simulink model "AutoParkFollowingBehaviour"  (R2023b)
settings: Solver=VariableStepAuto  StartTime=0  StopTime=2000  RelTol=1e-3
values from neighbouring files (symbols this model uses):
  simStepSize = 0.1    [AutoParkScenarioScript.m]
undefined symbols (not defined in the file or in its folder): Defined, Ego, Lane, User
libraries: roadrunnerscenario x3
settings Model: Creator=darkh  LastModifiedBy=varun

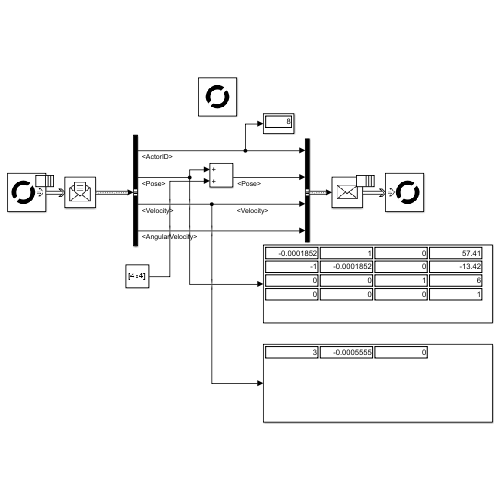
[thumbnail: Simulink's stored preview of the top-level diagram]
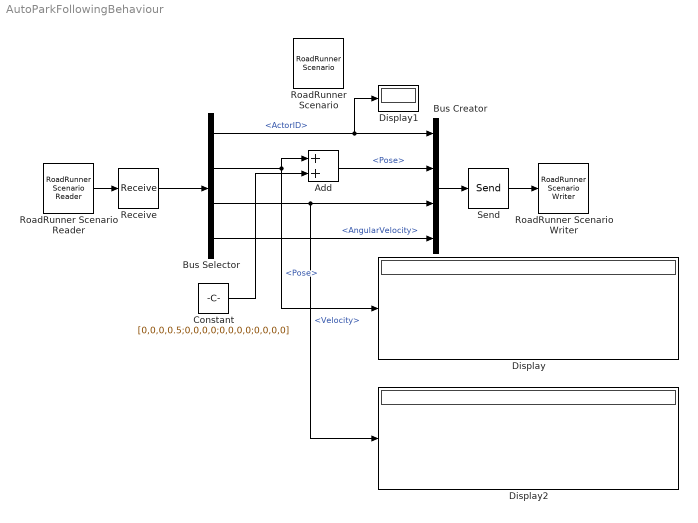
== system AutoParkFollowingBehaviour ==
  Add : Sum
  Bus Creator : BusCreator  Inputs=4  OutDataTypeStr=Bus: BusActorRuntime  NonVirtualBus=on
  Bus Selector : BusSelector  OutputSignals=ActorID,Pose,Velocity,AngularVelocity
  Constant : Constant  Value=[0,0,0,0.5;0,0,0,0;0,0,0,0;0,0,0,0]  SampleTime=simStepSize
  Display : Display
  Display1 : Display
  Display2 : Display
  Receive : Receive  InputPortMessageModes=m  UseInternalQueue=off  QueueOverwriting=on  QueueLength=1  QueueType=LIFO
  RoadRunner Scenario : roadrunnerscenario/RoadRunner Scenario  UserDefinedActions={}  UserDefinedEvents={}
  RoadRunner Scenario Reader : roadrunnerscenario/RoadRunner Scenario Reader  TopicCategory=Actor  ActorCategory=All Types  ActionType=Path Following  EventType=User-Defined  TopicType=Actor Pose  VehicleType=Vehicle Specifications  UserDefinedAction=Action1  UserDefinedEvent=Event1  Filter=Self  SensorTopic=Target Poses  LaneBoundaryOutputTopic=Ego-Lane  SensorID=1  SampleTime=simStepSize
  RoadRunner Scenario Writer : roadrunnerscenario/RoadRunner Scenario Writer  TopicCategory=Actor  ActorCategory=All Types  EventType=Action Complete  UserDefinedEvent=Event1  VehicleType=Vehicle Pose  TopicType=Actor Pose
  Send : Send  OutputPortMessageModes=m
  wires:
  Constant/1 -> Add/2
  Send/1 -> RoadRunner Scenario Writer/1
  Bus Selector/2 -> Display/1, Add/1  "<Pose>"
  RoadRunner Scenario Reader/1 -> Receive/1
  Bus Selector/1 -> Display1/1, Bus Creator/1  "<ActorID>"
  Bus Selector/3 -> Bus Creator/3, Display2/1  "<Velocity>"
  Bus Selector/4 -> Bus Creator/4  "<AngularVelocity>"
  Bus Creator/1 -> Send/1
  Receive/1 -> Bus Selector/1
  Add/1 -> Bus Creator/2  "<Pose>"
